simulink model "ModelLinearizePendulumRCSPlant"  (R2018b)
settings: Solver=VariableStepAuto  StartTime=0.0  StopTime=10.0  RelTol=1e-3
settings Model: Creator=mendicantbias  LastModifiedBy=mendicantbias

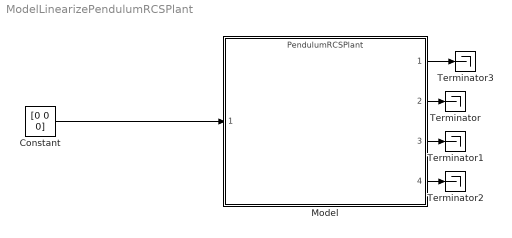
== system ModelLinearizePendulumRCSPlant ==
  Constant : Constant  Value=[0 0 0]
  Model : ModelReference  ModelNameDialog=PendulumRCSPlant  SimulationMode=Normal  ModelReferenceVersion=1.182
  Terminator{,1..3} (4 alike) : Terminator
  wires:
  Constant/1 -> Model/1
  Model/2 -> Terminator/1
  Model/3 -> Terminator1/1
  Model/4 -> Terminator2/1
  Model/1 -> Terminator3/1
